simulink library "SimMainLibrary"  (R2017b)
settings: Solver=ode45  StartTime=0.0  StopTime=10.0  RelTol=1e-3  EnableMultiTasking=on
values from neighbouring files (symbols this model uses):
  A = eye(16,16)    [full_input_list.m]
  B = zeros(16,1)    [full_input_list.m]
  C = blkdiag(eye(3,3),zeros(3,3),eye(10,10))    [full_input_list.m]
  centerMass = 2.7719    [full_input_list.m]
  H = C    [full_input_list.m]
  homeClock = clock    [full_input_list.m]    (also in initSimulink.m)
  kane_density = 1000    [full_input_list.m]
  m = 4*1/6    (= 0.666666666667)    [initACS.m]
  mewE = 3.986004418e14    (= 398600441800000)    [full_input_list.m]    (also in initACS.m)
  Q_k = zeros(16,16)    [full_input_list.m]
  R = R_k    [full_input_list.m]
  side1Dim = [ 10 10 6.124 ]/100    [full_input_list.m]
  side1Mass = 0.3283    [full_input_list.m]
  side2Dim = [ 10 10 6.124 ]/100    [full_input_list.m]
  st = 1/freq    (= 0.0125)    [full_input_list.m]    (also in initSimulink.m)
  state1_i = [ 0 0 0 , 0 0 0 , q4_0', w0_N]'    [full_input_list.m]
  state2_i = [ 0 0 (teth_length+side1Dim(1)/2+centerDim(3)/2+10*eps) , 0 -.1 0 ,      q4_0_Cube2' , w0_N ]'    [full_input_list.m]
  state3_i = [ 0 0 -(teth_length+side1Dim(1)/2+centerDim(3)/2+10*eps), 0 .1 0 ,      q4_0_Cube3' , w0_N ]'    [full_input_list.m]
  teth_length = 1    [full_input_list.m]
  teth_numLinks = 3    [full_input_list.m]
  u_k = zeros(16,1)    [full_input_list.m]
  w_k = zeros(16,1)    [full_input_list.m]
  Z_k = zeros(16,1)    [full_input_list.m]
undefined symbols (not defined in the file or in its folder): DiscIntNeverNeededParam, IAU, spring1kd, spring1ks, X, Y, Z
libraries: sm_lib x113, SimMainLibrary x27, nesl_utility x24, simulink x9, sharedutil x2, dspmtrx3 x1, dspinverses x1, aerolibtransform2 x1, aerolibgravity2 x1
(part 1 of 7)
settings Model: Creator=dtk42  LastModifiedBy=Aaron
settings DataIOCC: LimitDataPoints=on
settings OptimizationCC: LifeSpan=inf
settings DebuggingCC: AllowSymbolicDim=off  SFUnexpectedBacktrackingDiag=warning  SFNoUnconditionalDefaultTransitionDiag=warning  SFExecutionAtInitializationDiag=none
settings CodeAppCC: StateflowObjectComments=on
settings GRTTargetCC: TargetLangStandard=C89/C90 (ANSI)  GeneratePreprocessorConditionals=Disable all
settings ConfigComp: CovMetricSettings=dw  CovHtmlReporting=on  CovSaveCumulativeToWorkspaceVar=on  CovSaveSingleToWorkspaceVar=on  CovExternalEMLEnable=off

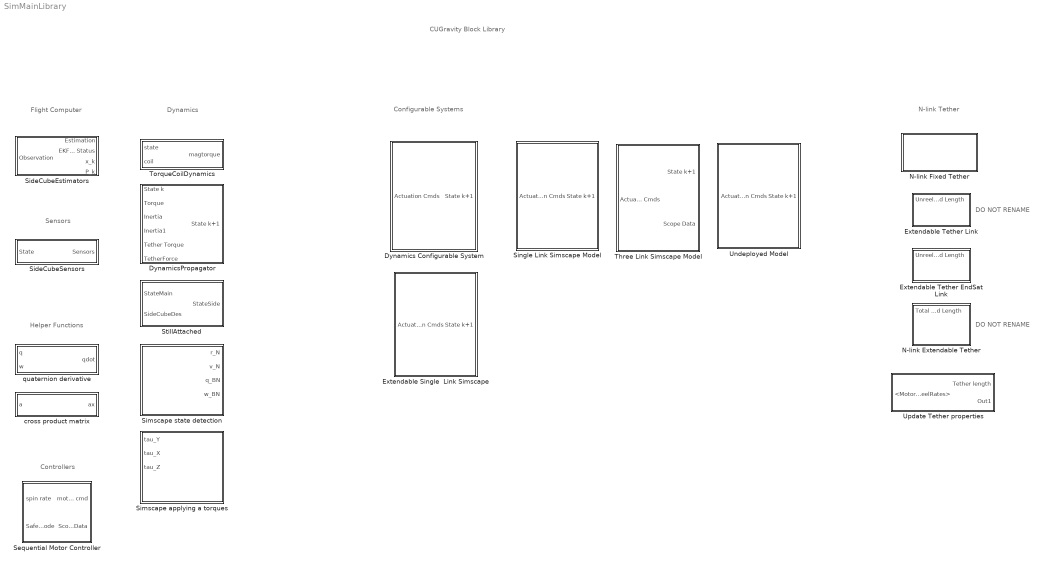
== system SimMainLibrary ==
  note: DO NOT RENAME
  note: N-link Tether
  note: Sensors
  note: CUGravity Block Library
  note: Flight Computer
  note: Dynamics
  note: Helper Functions
  note: Configurable Systems
  note: Controllers
  note: DO NOT RENAME
  Dynamics Configurable System : Subsystem  BlockChoice=Single Link Simscape Model
      settings: TemplateBlock=self  MemberBlocks="Extendable Single  Link Simscape ,Single Link Simscape Model,Three Link Simscape Model,Undeployed Model"
  DynamicsPropagator : Subsystem
  "Extendable Single  Link Simscape " : Subsystem
  Extendable Tether EndSat Link : Subsystem  AncestorBlock=SimMainLibrary/Extendable Tether Link
  Extendable Tether Link : Subsystem
  N-link Extendable Tether : Subsystem
  N-link Fixed Tether : Subsystem
  Sequential Motor Controller : Subsystem
  SideCubeEstimators : Subsystem
  SideCubeSensors : Subsystem
  Simscape applying a torques : Subsystem
  Simscape state detection : Subsystem
  Single Link Simscape Model : Subsystem
  StillAttached : Subsystem
  Three Link Simscape Model : Subsystem
  TorqueCoilDynamics : Subsystem
  Undeployed Model : Subsystem
  Update Tether properties : Subsystem
  cross product matrix : Subsystem
  quaternion derivative : Subsystem

== system SimMainLibrary/Dynamics Configurable System ==
  Actuation Cmds : Inport
  Single Link Simscape Model : SimMainLibrary/Single Link Simscape Model
      settings: SourceProductName=CUGravity Library
  State k+1 : Outport
  wires:
  Actuation Cmds/1 -> Single Link Simscape Model/1
  Single Link Simscape Model/1 -> State k+1/1

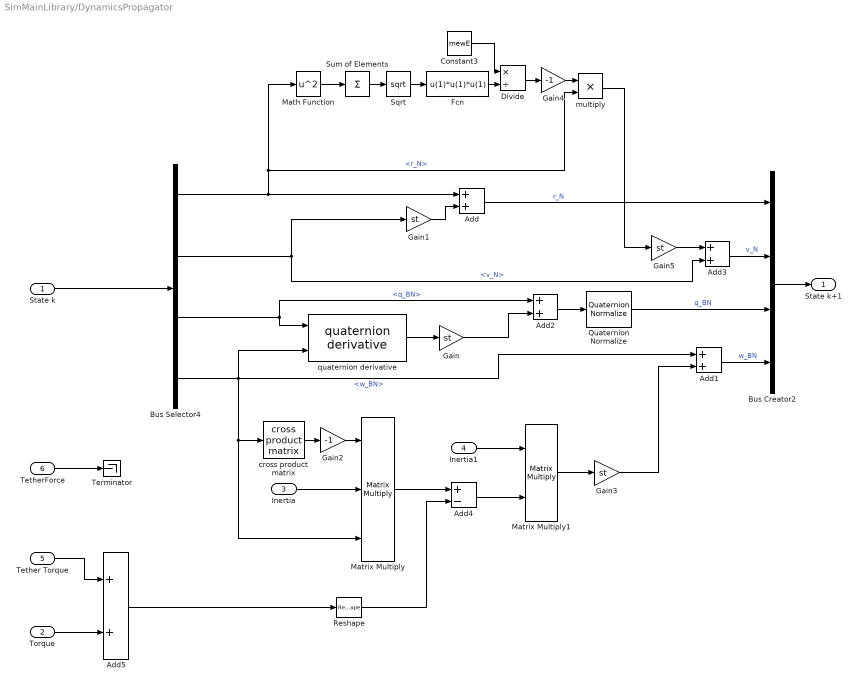
== system SimMainLibrary/DynamicsPropagator ==
  State k : Inport
  Torque : Inport  Port=2
  Inertia : Inport  Port=3
  Inertia1 : Inport  Port=4
  Tether Torque : Inport  Port=5
  TetherForce : Inport  Port=6
  Add{,1..3,5} (5 alike) : Sum
  Add4 : Sum  Inputs=+-
  Bus Creator2 : BusCreator  Inputs='r_N','v_N','q_BN','w_BN'
  Bus Selector4 : BusSelector  OutputSignals=r_N,v_N,q_BN,w_BN
  Constant3 : Constant  Value=mewE
  Divide : Product  Inputs=*/
  Fcn : Fcn  Expr=u(1)*u(1)*u(1)
  Gain{,1,3,5} (4 alike) : Gain  Gain=st
  Gain2 : Gain  Gain=-1
  Gain4 : Gain  Gain=-1
  Math Function : Math  Operator=square  SaturateOnIntegerOverflow=on
  Matrix Multiply : Product  Inputs=3  Multiplication=Matrix(*)
  Matrix Multiply1 : Product  Multiplication=Matrix(*)
  Quaternion Normalize : sharedutil/Quaternion Normalize
      settings: SourceProductName=Aerospace Blockset  SourceProductBaseCode=AE
  Reshape : Reshape  OutputDimensionality=Column vector (2-D)
  Sqrt : Sqrt  SaturateOnIntegerOverflow=on
  Sum of Elements : Sum  Inputs=+
  Terminator : Terminator
  cross product matrix : SimMainLibrary/cross product matrix
      settings: SourceProductName=CUGravity Library
  multiply : Product  Inputs=**
  quaternion derivative : SimMainLibrary/quaternion derivative
      settings: SourceProductName=CUGravity Library
  State k+1 : Outport
  wires:
  Quaternion Normalize/1 -> Bus Creator2/3  "q_BN"
  Math Function/1 -> Sum of Elements/1
  Bus Selector4/3 -> Add2/1, quaternion derivative/1  "<q_BN>"
  Gain5/1 -> Add3/1
  Sqrt/1 -> Fcn/1
  Bus Selector4/1 -> multiply/2, Math Function/1, Add/1  "<r_N>"
  Gain2/1 -> Matrix Multiply/1
  Bus Selector4/4 -> Matrix Multiply/3, cross product matrix/1, Add1/1, quaternion derivative/2  "<w_BN>"
  quaternion derivative/1 -> Gain/1
  Sum of Elements/1 -> Sqrt/1
  Gain4/1 -> multiply/1
  multiply/1 -> Gain5/1
  Gain3/1 -> Add1/2
  State k/1 -> Bus Selector4/1
  Bus Selector4/2 -> Gain1/1, Add3/2  "<v_N>"
  Gain/1 -> Add2/2
  Add1/1 -> Bus Creator2/4  "w_BN"
  Add2/1 -> Quaternion Normalize/1
  Add3/1 -> Bus Creator2/2  "v_N"
  Inertia/1 -> Matrix Multiply/2
  cross product matrix/1 -> Gain2/1
  Bus Creator2/1 -> State k+1/1
  Gain1/1 -> Add/2
  Add4/1 -> Matrix Multiply1/2
  Matrix Multiply1/1 -> Gain3/1
  Matrix Multiply/1 -> Add4/1
  Fcn/1 -> Divide/2
  Divide/1 -> Gain4/1
  Add/1 -> Bus Creator2/1  "r_N"
  Constant3/1 -> Divide/1
  TetherForce/1 -> Terminator/1
  Tether Torque/1 -> Add5/1
  Torque/1 -> Add5/2
  Add5/1 -> Reshape/1
  Inertia1/1 -> Matrix Multiply1/1
  Reshape/1 -> Add4/2
